simulink model "Phase 1 Energy modelling-BMW i4 eDrive35 Gran Coupe Simulation"  (R2025b)
settings: Solver=VariableStepAuto  StartTime=0  StopTime=1369  RelTol=1e-3  AbsTol=1e-3
libraries: fl_lib x11, nesl_utility x6, sdl_lib x4, autolibshared x2, ee_lib x1
settings Model: Creator=abbaskhanian.k  LastModifiedBy=kunas
settings SolverCC: AutoScaleAbsTol=off  AlgebraicLoopSolver=TrustRegion
settings DebuggingCC: UnconnectedInputMsg=warning  UnconnectedOutputMsg=warning  UnconnectedLineMsg=warning  SymbolicDimsDataTypeCodeGenerationDiagnostic=none
settings ModelReferenceCC: EnableRefExpFcnMdlSchedulingChecks=on
settings SFSimCC: CustomCodeUndefinedFunction=UseInterfaceOnly
settings RTWCC: GPUComputeCapability=3.5  DLArmComputeVersion=19.05
settings SimscapeCC: SimscapeLogType=all  SimscapeLogSimulationStatistics=on  SimscapeLogDataHistory=10000.0

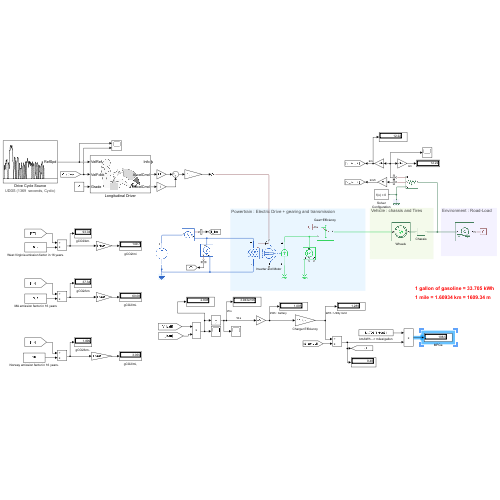
[thumbnail: Simulink's stored preview of the top-level diagram]
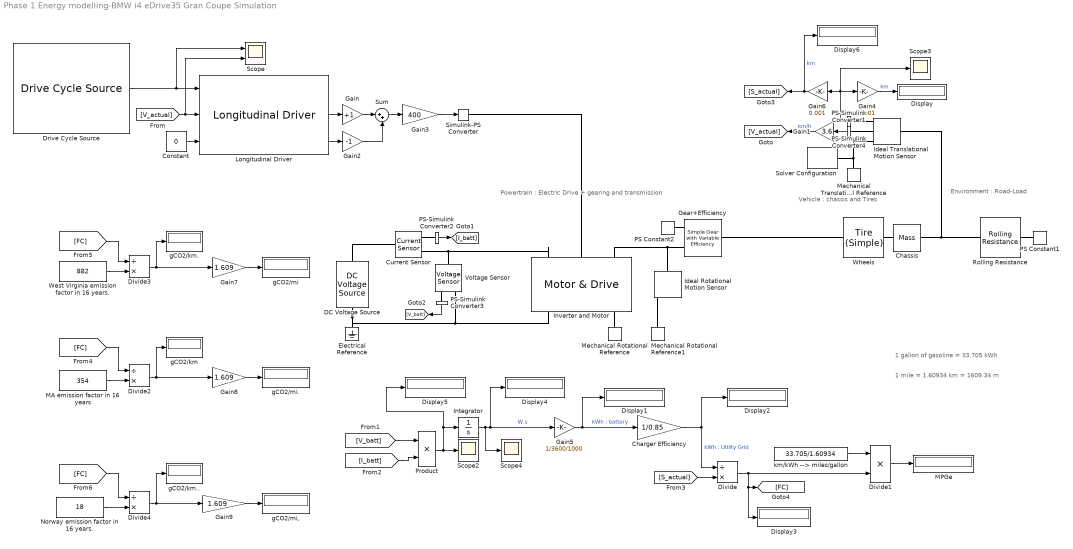
== system Phase 1 Energy modelling-BMW i4 eDrive35 Gran Coupe Simulation ==
  note: 1 gallon of gasoline = 33.705 kWh
  note: Powertrain : Electric Drive + gearing and transmission
  note: Vehicle : chassis and Tires
  note: Environment : Road-Load
  note: 1 mile = 1.60934 km = 1609.34 m
  Charger Efficiency : Gain  Gain=1/0.85
  Chassis : fl_lib/Mechanical/Translational Elements/Mass  mass=1970 kg  num_ports=foundation.enum.numPorts2.two  v_specify=off  v_priority=High  v=0 m/s  v_nominal_specify=off  v_nominal_value=1  v_nominal_unit=m/s  f_specify=off  f_priority=None  f=0 N  f_nominal_specify=off  f_nominal_value=1  f_nominal_unit=N
      settings: InternalSimscapePortConfiguration="{\"Bottom\":[],\"Left\":[{\"id\":\"M\",\"label\":\"\",\"type\":\"foundation.mechanical.translational.translational\"}],\"Right\":[{\"id\":\"N\",\"label\":\"\",\"type\":\"foundation.mechanical.translational.translational\"}],\"Top\":[]}"
  Constant : Constant  Value=0
  Current Sensor : fl_lib/Electrical/Electrical Sensors/Current Sensor
  DC Voltage Source : ee_lib/Additional Components/SPICE Sources/DC Voltage Source  DC=400 V
  Display{,1..6} (7 alike) : Display
  Divide{,2..4} (4 alike) : Product  Inputs=/*
  Divide1 : Product  Inputs=**
  Drive Cycle Source : autolibshared/Drive Cycle Source  cycleVar=UDDS  fileVar=cycleFTP75.mat  tfinal="1369  seconds, Cyclic"  cycleRepeat=on  outAccPort=off  outGearPort=off  gearList=No gear data  t_wot1=5  xdot_woto=0  xdot_wot1=30  t_wot2=20  xdot_wot2=0  t_wotend=30  srcUnit=m/s  outUnit=km/h  srcAccUnit=m/s/s  outAccUnit=m/s^2  dt=0  aMode=1  faultOption=off  velBnd=2  velBndUnit=mph  inUnit=m/s  timeBnd=1  failOption=off  stopSim=off  maxFaultCnt=10  maxFaultTime=2  maxTotFaultTime=15  traceOption=off  dtTrace=1  traceWindow=10  lastDCname=UDDS  lastOutUnit=mph  lastDT=0  lastTB=1  lastSB=2  forceCalcBound=off
  Electrical Reference : fl_lib/Electrical/Electrical Elements/Electrical Reference
  Gain : Gain  Gain=+1
  Gain1 : Gain  Gain=3.6
  Gain2 : Gain  Gain=-1
  Gain3 : Gain  Gain=400
  Gain4 : Gain  Gain=0.001
  Gain5 : Gain  Gain=1/3600/1000
  Gain6 : Gain  Gain=0.001
  Gain7 : Gain  Gain=1.609
  Gain8 : Gain  Gain=1.609
  Gain9 : Gain  Gain=1.609
  "Gear+Efficiency " : sdl_lib/Gears/Simple Gear with Variable Efficiency  ratio=8.77  rotation_direction=sdl.enum.shaftOutputDirection.same  min_efficiency=0.96  pwr_thr=50 W  mu_visc=[0, 0] N*m/(rad/s)  thermal_port=simscape.enum.thermaleffects.omit  thermal_mass=50 J/K  temperature_specify=off  temperature_priority=High  temperature=300 K  temperature_nominal_specify=off  temperature_nominal_value=1  temperature_nominal_unit=K
      settings: InternalSimscapePortConfiguration="{\"Bottom\":[],\"Left\":[{\"id\":\"E\",\"label\":\"E\",\"type\":\"input\"},{\"id\":\"B\",\"label\":\"B\",\"type\":\"foundation.mechanical.rotational.rotational\"}],\"Right\":[{\"id\":\"F\",\"label\":\"F\",\"type\":\"foundation.mechanical.rotational.rotational\"}],\"Top\":[]}"
  Ideal Rotational Motion Sensor : fl_lib/Mechanical/Mechanical Sensors/Ideal Rotational Motion Sensor  reference=foundation.enum.MeasurementReference.difference  acceleration_port=false  velocity_port=true  position_port=true  wrap_angle=simscape.enum.onoff.off  offset=0 rad
  Ideal Translational Motion Sensor : fl_lib/Mechanical/Mechanical Sensors/Ideal Translational Motion Sensor  reference=foundation.enum.MeasurementReference.difference  acceleration_port=false  velocity_port=true  position_port=true  offset=0 m
  Integrator : Integrator
  Inverter and Motor : sdl_lib/Engines & Motors/Motor & Drive  torque_max=400 N*m  power_max=210 kW  Tc=0.03 s  eff=85  w_eff=2000 rpm  T_eff=100 N*m  thermal_port=simscape.enum.thermaleffects.omit  thermal_mass=100 J/K  temperature_specify=off  temperature_priority=High  temperature=300 K  temperature_nominal_specify=off  temperature_nominal_value=1  temperature_nominal_unit=K
      settings: InternalSimscapePortConfiguration="{\"Bottom\":[],\"Left\":[{\"id\":\"Vp\",\"label\":\"+\",\"type\":\"foundation.electrical.electrical\"},{\"id\":\"Tr\",\"label\":\"Tr\",\"type\":\"input\"},{\"id\":\"R\",\"label\":\"R\",\"type\":\"foundation.mechanical.rotational.rotational\"}],\"Right\":[{\"id\":\"Vm\",\"label\":\"-\",\"type\":\"foundation.electrical.electrical\"},{\"id\":\"Omega\",\"label\":\"w\",\"type\":\"output\"},{\"id\":\"C\",\"label\":\"C\",\"type\":\"foundation.mechanical.rotational.rotational\"}],\"Top\":[]}"
  Longitudinal Driver : autolibshared/Longitudinal Driver  extAccelOvr=off  extDecelOvr=off  extAccelHld=off  extDecelHld=off  extAccelZero=off  extDecelZero=off  cntrlType=PI  shftType=None  velUnits=km/h  gearOut=off  Kp=1  Ki=5  Kff=.05  Kg=.01  VehVelVec=[0 100]  KffVec=[.1 .1]  KpVec=[10 10]  KiVec=[5 5]  KgVec=[0 0]  m=1500  Kpt=3000  tau=.1  L=2  aR=200  bR=2.5  cR=.5  g=9.81  vnom=120  Kaw=.5  tauerr=.1  tauPt=2  GearInit=0  tShift=.1  pdlVec=[0.1 0.4 0.5 0.9]  upShftTbl=[-1 12.9375 26.4375 39.9375 51.18749999999999 62.4375 72.84375 83.25;-1 16.3125 29.8125 43.3125 54.5624 65.8125 76.78125 87.75;-1 19.6875 33.1875 46.68749999999999 57.9375 69.1875 80.71875 92.25;-1 33 52.5 77.25 100.5 138.75 161.875 185]  dwnShftTbl=[1 9.5625 23.0625 36.5625 47.8125 59.0625 68.90625 78.75;1 12.9375 26.4375 39.9375 51.18749999999999 62.4375 72.84375 83.25;1 16.3125 29.8125 43.3125 54.562499 65.8125 76.78125 87.75;1 19.6875 33.1875 46.68749999999999 57.9375 69.1875 80.71875 92.25]  tClutch=.5  tRev=.5  tPark=120  aMode=1  UpGearVec="[0  1  2  3  4  5  6  7]"  DownGearVec="[1  2  3  4  5  6  7  8]"
  MA emission factor in 16 years : Constant  Value=354
  MPGe : Display
  Mechanical Rotational Reference : fl_lib/Mechanical/Rotational Elements/Mechanical Rotational Reference
  Mechanical Rotational Reference1 : fl_lib/Mechanical/Rotational Elements/Mechanical Rotational Reference
  Mechanical Translational Reference : fl_lib/Mechanical/Translational Elements/Mechanical Translational Reference
  Norway emission factor in 16 years. : Constant  Value=18
  PS Constant1 : fl_lib/Physical Signals/Sources/PS Constant  constant=1
  PS Constant2 : fl_lib/Physical Signals/Sources/PS Constant  constant=0.96
  PS-Simulink Converter{1..4} (4 alike) : nesl_utility/PS-Simulink Converter  PhysicalDomain=network_engine_domain  SubClassName=ps_output  LeftPortType=input  RightPortType=output  PseudoPeriodic=off  Frequencies=[]  VectorFormat=1-D array  Unit=inherit  AffineConversion=off
  Product : Product
  Rolling Resistance : sdl_lib/Tires & Vehicles/Tire Subcomponents/Rolling Resistance  model=sdl.enum.rollingResistanceParameterization.velocity  coeff=0.015  p_tire=269e3 Pa  alpha=0  beta=0  coeff_a=141.9  coeff_b=0.299 s/m  coeff_c=0.360 s^2/m^2  p_tire0=240e3 Pa  fz0=4000 N  vH0=16 m/s  q_Sy=[.0082, 0, .0014, .001, 0, 0, 1.08, -.5]  lmy=1  v_thr=1 m/s
      settings: InternalSimscapePortConfiguration="{\"Bottom\":[],\"Left\":[{\"id\":\"N\",\"label\":\"N\",\"type\":\"input\"}],\"Right\":[{\"id\":\"H\",\"label\":\"H\",\"type\":\"foundation.mechanical.translational.translational\"}],\"Top\":[]}"
  Scope : Scope  NumInputPorts=2
      settings: ActiveDisplayYMinimum=-12.789883505004171  ActiveDisplayYMaximum=103.30913108816584
  Scope2 : Scope
      settings: ActiveDisplayYMinimum=-1  ActiveDisplayYMaximum=1  DataLoggingVariableName=ScopeData2
  Scope3 : Scope
      settings: ActiveDisplayYMinimum=-2227.52679069337  ActiveDisplayYMaximum=20047.741116240333  DataLoggingVariableName=ScopeData3
  Scope4 : Scope
      settings: ActiveDisplayYMinimum=-785296.49807  ActiveDisplayYMaximum=7.06766848259E+6  DataLoggingVariableName=ScopeData4
  Simulink-PS Converter : nesl_utility/Simulink-PS Converter  PhysicalDomain=network_engine_domain  SubClassName=ps_input  LeftPortType=input  RightPortType=output  PseudoPeriodic=off  Frequencies=[]  NoiseDistribution=none  NoiseParameters=[]  Unit=1  AffineConversion=off  FilteringAndDerivatives=provide  SimscapeFilterOrder=1  InputFilterTimeConstant=0.001  UdotUserProvided=0
  Solver Configuration : nesl_utility/Solver Configuration  PhysicalDomain=network_engine_domain  SubClassName=solver  LeftPortType=input  RightPortType=generic  Tones=[]  Harmonics=[]  SimulateNoise=off  Profile=off  UseLocalSampling=off  EnableSwitchedLinearOptims=on  FrequencyDomain=off  UseCCode=off  RelTol=0.001  AbsTol=1e-06  MinStep=1e-09  ToWorkspace=off  RevertToSquareIcSolve=off  NumHomotopyIterations=100  PhasorMode=off  PhasorModeNumHarmonics=1  ConsistencySolver=NEWTON_FTOL  IndexReductionMethod=DerivativeReplacement  DoDC=off  ResidualTolerance=1e-09  ConsistencyTolSource=GLOBAL  ConsistencyAbsTol=0.001  ConsistencyRelTol=0.001  ConsistencyTolFactor=0.001  UseLocalSolver=off  LocalSolverChoice=NE_BACKWARD_EULER_ADVANCER  ResolveIndetEquations=on  FunctionEvalNumThread=1  LocalSolverSampleTime=0.001  DoFixedCost=off  MaxNonlinIter=3  MaxModeIter=2  ComputeImpulses=off  ImpulseIterations=2  LinearAlgebra=auto  LinearAlgebraNumThread=0  EquationFormulation=NE_TIME_EF  DelaysMemoryBudget=1024  AutomaticFiltering=on  FilteringTimeConstant=0.001  PartitionStorageMethod=AS_NEEDED  PartitionMemoryBudget=1024  PartitionMethod=ROBUST  MultibodyUseLocalSolver=off  MultibodyLocalSolverChoice=ODE1  MultibodyLocalSolverSampleTime=0.001
  Sum : Sum  Inputs=|++
  Voltage Sensor : fl_lib/Electrical/Electrical Sensors/Voltage Sensor
  West Virginia emission factor in 16 years. : Constant  Value=882
  Wheels : sdl_lib/Tires & Vehicles/Tire (Simple)  r_tire=0.2286 m  model_compliance=sdl.enum.compliance.off  stiffness=1e6 N/m  damping=1000 N/(m/s)  model_inertia=sdl.enum.model_inertia.on  tire_inertia=1 kg*m^2  initial_velocity=0 rad/s
      settings: InternalSimscapePortConfiguration="{\"Bottom\":[],\"Left\":[{\"id\":\"A\",\"label\":\"A\",\"type\":\"foundation.mechanical.rotational.rotational\"}],\"Right\":[{\"id\":\"H\",\"label\":\"H\",\"type\":\"foundation.mechanical.translational.translational\"}],\"Top\":[]}"
  gCO2/km : Display
  gCO2/km. : Display
  gCO2/km.. : Display
  gCO2/mi : Display
  gCO2/mi, : Display
  gCO2/mi. : Display
  km/kWh --> miles/gallon : Constant  Value=33.705/1.60934
  wires:
  PS-Simulink Converter1/1 -> Gain1/1
  Gain1/1 -> [V_actual]  "km/h"
  Drive Cycle Source/1 -> Scope/1, Longitudinal Driver/1
  [V_actual] -> Scope/2, Longitudinal Driver/2
  Constant/1 -> Longitudinal Driver/3
  Longitudinal Driver/2 -> Gain/1
  Longitudinal Driver/3 -> Gain2/1
  Gain/1 -> Sum/1
  Gain2/1 -> Sum/2
  Sum/1 -> Gain3/1
  PS-Simulink Converter3/1 -> [V_batt]
  [I_batt] -> Product/2
  [V_batt] -> Product/1
  Product/1 -> Scope2/1, Integrator/1, Display5/1
  PS-Simulink Converter4/1 -> Gain4/1, Gain6/1, Scope3/1
  Integrator/1 -> Gain5/1, Display4/1, Scope4/1  "W.s"
  Gain4/1 -> Display/1  "km"
  Gain5/1 -> Charger Efficiency/1, Display1/1  "kWh : battery"
  Gain6/1 -> Display6/1, [S_actual]  "km"
  [S_actual] -> Divide/2
  Divide/1 -> Display3/1, [FC], Divide1/2
  km/kWh --> miles/gallon/1 -> Divide1/1
  Divide1/1 -> MPGe/1
  Charger Efficiency/1 -> Divide/1, Display2/1  "kWh : Utility Grid"
  PS-Simulink Converter2/1 -> [I_batt]
  Gain3/1 -> Simulink-PS Converter/1
  Divide2/1 -> gCO2/km/1, Gain8/1
  MA emission factor in 16 years/1 -> Divide2/2
  [FC] -> Divide2/1
  Divide3/1 -> Gain7/1, gCO2/km./1
  [FC] -> Divide3/1
  West Virginia emission factor in 16 years./1 -> Divide3/2
  Divide4/1 -> Gain9/1, gCO2/km../1
  Norway emission factor in 16 years./1 -> Divide4/2
  [FC] -> Divide4/1
  Gain7/1 -> gCO2/mi/1
  Gain8/1 -> gCO2/mi./1
  Gain9/1 -> gCO2/mi,/1
  connections:
  Mechanical Rotational Reference/LConn1 -- Inverter and Motor/RConn3
  "Gear+Efficiency "/LConn2 -- Ideal Rotational Motion Sensor/LConn1 -- Inverter and Motor/LConn3
  Wheels/RConn1 -- Chassis/LConn1
  Wheels/LConn1 -- "Gear+Efficiency "/RConn1
  Rolling Resistance/RConn1 -- Ideal Translational Motion Sensor/LConn1 -- Chassis/RConn1
  PS Constant1/RConn1 -- Rolling Resistance/LConn1
  Ideal Translational Motion Sensor/RConn1 -- Solver Configuration/RConn1 -- Mechanical Translational Reference/LConn1
  Ideal Translational Motion Sensor/RConn2 -- PS-Simulink Converter1/LConn1
  Inverter and Motor/LConn2 -- Simulink-PS Converter/RConn1
  Ideal Rotational Motion Sensor/RConn1 -- Mechanical Rotational Reference1/LConn1
  PS Constant2/RConn1 -- "Gear+Efficiency "/LConn1
  DC Voltage Source/LConn1 -- Current Sensor/LConn1
  DC Voltage Source/RConn1 -- Inverter and Motor/RConn1 -- Voltage Sensor/RConn2 -- Electrical Reference/LConn1
  PS-Simulink Converter2/LConn1 -- Current Sensor/RConn1
  PS-Simulink Converter3/LConn1 -- Voltage Sensor/RConn1
  Inverter and Motor/LConn1 -- Current Sensor/RConn2 -- Voltage Sensor/LConn1
  PS-Simulink Converter4/LConn1 -- Ideal Translational Motion Sensor/RConn3
